simulink model "rhombus_vehicle_model_github"  (R2025b)
settings: Solver=VariableStepAuto  StartTime=0.0  StopTime=10.0  RelTol=1e-3
values from neighbouring files (symbols this model uses):
  B = 0.865    [vehicle_params_github.m]
  Bphi = 1.2e5    (= 120000)    [vehicle_params_github.m]
  Bx = 2    [vehicle_params_github.m]
  By = 1.5    [vehicle_params_github.m]
  Cw = 5    [vehicle_params_github.m]
  Cx = 1.1    [vehicle_params_github.m]
  Cy = 1.1    [vehicle_params_github.m]
  Ex = 0.3    [vehicle_params_github.m]
  Ey = -1.0    (= -1)    [vehicle_params_github.m]
  g = 9.81    [vehicle_params_github.m]
  hs = 1.25    [vehicle_params_github.m]
  Ix = 7.5e4    (= 75000)    [vehicle_params_github.m]
  Ixz = 0    [vehicle_params_github.m]
  Iz = 2.5e6    (= 2500000)    [vehicle_params_github.m]
  Jw = 60    [vehicle_params_github.m]
  kphi = 8e5    (= 800000)    [vehicle_params_github.m]
  lf = 4    [vehicle_params_github.m]
  lm = 0    [vehicle_params_github.m]
  lr = 4    [vehicle_params_github.m]
  m = 28000    [vehicle_params_github.m]
  ms = 22000    [vehicle_params_github.m]
  mux = 0.3    [vehicle_params_github.m]
  muy = 0.6    [vehicle_params_github.m]
  p = -0.15    [vehicle_params_github.m]
  Rw = 0.5    [vehicle_params_github.m]
settings Model: Creator=dastiw  LastModifiedBy=dastiw

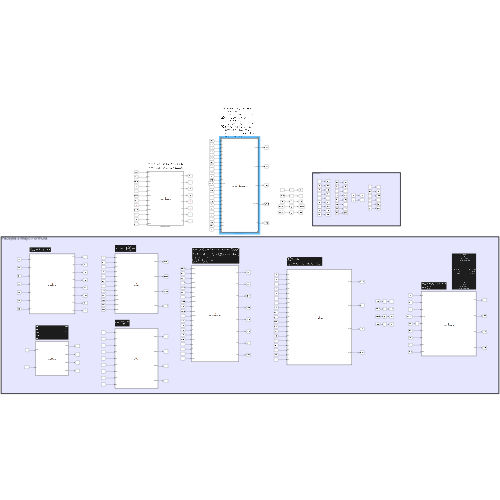
[thumbnail: Simulink's stored preview of the top-level diagram]
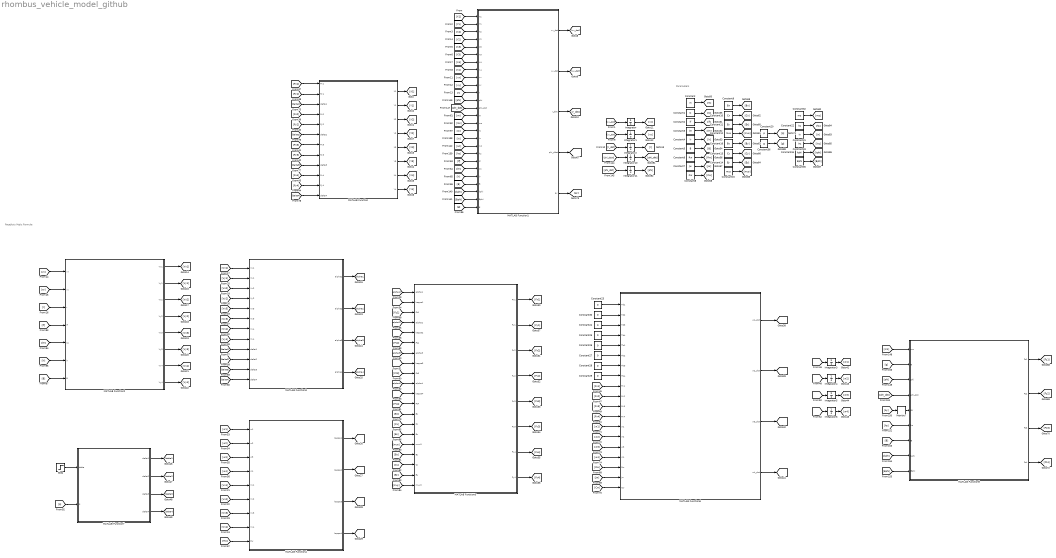
== system rhombus_vehicle_model_github ==
  note: Pacejka's Majic Formula
  note: Parameters
  Constant : Constant  Value=m
  Constant1 : Constant  Value=Iz
  Constant10 : Constant  Value=Cx
  Constant11 : Constant  Value=Ex
  Constant12 : Constant  Value=mux
  Constant13 : Constant  Value=Cy
  Constant14 : Constant  Value=Ey
  Constant15 : Constant  Value=muy
  Constant16 : Constant  Value=By
  Constant2 : Constant  Value=lf
  Constant20 : Constant  Value=p
  Constant22 : Constant  Value=hs
  Constant{23..30} (8 alike) : Constant  Value=0
  Constant3 : Constant  Value=lm
  Constant31 : Constant  Value=Ix
  Constant32 : Constant  Value=ms
  Constant33 : Constant  Value=Ixz
  Constant34 : Constant  Value=kphi
  Constant35 : Constant  Value=Bphi
  Constant36 : Constant  Value=g
  Constant4 : Constant  Value=lr
  Constant5 : Constant  Value=B
  Constant6 : Constant  Value=Rw
  Constant7 : Constant  Value=Jw
  Constant8 : Constant  Value=Cw
  Constant9 : Constant  Value=Bx
  Integrator : Integrator  InitialCondition=5
  Integrator{1..2,10..11} (4 alike) : Integrator
  Integrator{3..6} (4 alike) : Integrator  InitialCondition=5/Rw
  MATLAB Function : MATLAB Function  TreatAsAtomicUnit=on
  MATLAB Function1 : MATLAB Function  TreatAsAtomicUnit=on
  MATLAB Function2 : MATLAB Function  TreatAsAtomicUnit=on
  MATLAB Function3 : MATLAB Function  TreatAsAtomicUnit=on
  MATLAB Function4 : MATLAB Function  TreatAsAtomicUnit=on
  MATLAB Function5 : MATLAB Function  TreatAsAtomicUnit=on
  MATLAB Function6 : MATLAB Function  TreatAsAtomicUnit=on
  MATLAB Function7 : MATLAB Function  TreatAsAtomicUnit=on
  MATLAB Function9 : MATLAB Function  TreatAsAtomicUnit=on
  Memory : Memory
  Step : Step  After=0.01  SampleTime=0
  wires:
  MATLAB Function/1(X1) -> [X1]
  MATLAB Function/8(Y4) -> [Y4]
  MATLAB Function/2(Y1) -> [Y1]
  MATLAB Function/3(X2) -> [X2]
  MATLAB Function/4(Y2) -> [Y2]
  MATLAB Function/5(X3) -> [X3]
  MATLAB Function/6(Y3) -> [Y3]
  MATLAB Function/7(X4) -> [X4]
  MATLAB Function1/1(vx_dot) -> [vx_dot]
  MATLAB Function1/2(vy_dot) -> [vy_dot]
  MATLAB Function1/3(r_dot) -> [r_dot]
  [vx_dot] -> Integrator/1
  [vy_dot] -> Integrator1/1
  [r_dot] -> Integrator2/1
  Integrator/1 -> [vx]
  Integrator1/1 -> [vy]
  Integrator2/1 -> [r]
  [vy] -> MATLAB Function2/2(vy)
  [vx] -> MATLAB Function2/1(vx)
  [r] -> MATLAB Function2/3(r)
  MATLAB Function2/1(Vx1) -> [Vx1]
  MATLAB Function2/3(Vx2) -> [Vx2]
  MATLAB Function2/5(Vx3) -> [Vx3]
  MATLAB Function2/7(Vx4) -> [Vx4]
  [Vx1] -> MATLAB Function3/1(Vx1)
  [Vx2] -> MATLAB Function3/3(Vx2)
  [Vx3] -> MATLAB Function3/5(Vx3)
  [Vx4] -> MATLAB Function3/7(Vx4)
  [Vx1] -> MATLAB Function4/5(Vx1)
  [Vx4] -> MATLAB Function4/8(Vx4)
  [Vx3] -> MATLAB Function4/7(Vx3)
  [Vx2] -> MATLAB Function4/6(Vx2)
  MATLAB Function2/2(Vy1) -> [Vy1]
  MATLAB Function2/4(Vy2) -> [Vy2]
  MATLAB Function2/6(Vy3) -> [Vy3]
  MATLAB Function2/8(Vy4) -> [Vy4]
  [Vy1] -> MATLAB Function3/2(Vy1)
  [Vy2] -> MATLAB Function3/4(Vy2)
  [Vy3] -> MATLAB Function3/6(Vy3)
  [Vy4] -> MATLAB Function3/8(Vy4)
  MATLAB Function3/1(alpha1) -> [alpha1]
  MATLAB Function3/2(alpha2) -> [alpha2]
  MATLAB Function3/3(alpha3) -> [alpha3]
  MATLAB Function3/4(alpha4) -> [alpha4]
  MATLAB Function4/1(kappa1) -> [kappa1]
  MATLAB Function4/2(kappa2) -> [kappa2]
  MATLAB Function4/3(kappa3) -> [kappa3]
  MATLAB Function4/4(kappa4) -> [kappa4]
  [alpha1] -> MATLAB Function5/1(alpha1)
  [kappa1] -> MATLAB Function5/2(kappa1)
  [alpha2] -> MATLAB Function5/4(alpha2)
  [kappa2] -> MATLAB Function5/5(kappa2)
  [alpha3] -> MATLAB Function5/7(alpha3)
  [kappa3] -> MATLAB Function5/8(kappa3)
  [alpha4] -> MATLAB Function5/10(alpha4)
  [kappa4] -> MATLAB Function5/11(kappa4)
  MATLAB Function5/1(Fx1) -> [Fx1]
  MATLAB Function5/2(Fy1) -> [Fy1]
  MATLAB Function5/3(Fx2) -> [Fx2]
  MATLAB Function5/4(Fy2) -> [Fy2]
  MATLAB Function5/5(Fx3) -> [Fx3]
  MATLAB Function5/6(Fy3) -> [Fy3]
  MATLAB Function5/7(Fx4) -> [Fx4]
  MATLAB Function5/8(Fy4) -> [Fy4]
  [Fx1] -> MATLAB Function/1(Fx1)
  [Fy1] -> MATLAB Function/2(Fy1)
  [Fx2] -> MATLAB Function/4(Fx2)
  [Fy2] -> MATLAB Function/5(Fy2)
  [Fx3] -> MATLAB Function/7(Fx3)
  [Fy3] -> MATLAB Function/8(Fy3)
  [Fx4] -> MATLAB Function/10(Fx4)
  [Fy4] -> MATLAB Function/11(Fy4)
  [Fx1] -> MATLAB Function6/9(Fx1)
  [Fx2] -> MATLAB Function6/10(Fx2)
  [Fx3] -> MATLAB Function6/11(Fx3)
  [Fx4] -> MATLAB Function6/12(Fx4)
  MATLAB Function6/1(w1_dot) -> [w1_dot]
  MATLAB Function6/2(w2_dot) -> [w2_dot]
  MATLAB Function6/3(w3_dot) -> [w3_dot]
  MATLAB Function6/4(w4_dot) -> [w4_dot]
  [w1_dot] -> Integrator3/1
  [w4_dot] -> Integrator6/1
  [w3_dot] -> Integrator5/1
  [w2_dot] -> Integrator4/1
  Integrator3/1 -> [w1]
  Integrator6/1 -> [w4]
  Integrator5/1 -> [w3]
  Integrator4/1 -> [w2]
  [w1] -> MATLAB Function4/1(w1)
  [w2] -> MATLAB Function4/2(w2)
  [w3] -> MATLAB Function4/3(w3)
  [w4] -> MATLAB Function4/4(w4)
  MATLAB Function7/1(delta1) -> [delta1]
  MATLAB Function7/2(delta2) -> [delta2]
  MATLAB Function7/3(delta3) -> [delta3]
  MATLAB Function7/4(delta4) -> [delta4]
  [delta1] -> MATLAB Function3/9(delta1)
  [delta2] -> MATLAB Function3/10(delta2)
  [delta3] -> MATLAB Function3/11(delta3)
  [delta4] -> MATLAB Function3/12(delta4)
  [Rw] -> MATLAB Function4/9(Rw)
  [Rw] -> MATLAB Function6/17(Rw)
  [Cw] -> MATLAB Function6/19(Cw)
  [Jw] -> MATLAB Function6/18(Jw)
  [w3] -> MATLAB Function6/15(w3)
  [w2] -> MATLAB Function6/14(w2)
  [w1] -> MATLAB Function6/13(w1)
  [w4] -> MATLAB Function6/16(w4)
  [delta1] -> MATLAB Function/3(delta1)
  [delta2] -> MATLAB Function/6(delta2)
  [delta4] -> MATLAB Function/12(delta4)
  [delta3] -> MATLAB Function/9(delta3)
  [Bx] -> MATLAB Function5/13(Bx)
  [Cx] -> MATLAB Function5/14(Cx)
  [Ex] -> MATLAB Function5/15(Ex)
  [mux] -> MATLAB Function5/16(mux0)
  [By] -> MATLAB Function5/17(By)
  [Cy] -> MATLAB Function5/18(Cy)
  [Ey] -> MATLAB Function5/19(Ey)
  [muy] -> MATLAB Function5/20(muy0)
  [B] -> MATLAB Function2/7(B)
  [Fz1] -> MATLAB Function5/3(Fz1)
  [Fz2] -> MATLAB Function5/6(Fz2)
  [Fz3] -> MATLAB Function5/9(Fz3)
  [Fz4] -> MATLAB Function5/12(Fz4)
  [p] -> MATLAB Function7/2(p)
  [lf] -> MATLAB Function2/4(lf)
  [lm] -> MATLAB Function2/5(lm)
  [lr] -> MATLAB Function2/6(lr)
  Constant23/1 -> MATLAB Function6/1(Td1)
  Constant29/1 -> MATLAB Function6/8(Tb4)
  Constant28/1 -> MATLAB Function6/7(Tb3)
  Constant27/1 -> MATLAB Function6/6(Tb2)
  Constant26/1 -> MATLAB Function6/5(Tb1)
  Constant25/1 -> MATLAB Function6/4(Td4)
  Constant24/1 -> MATLAB Function6/3(Td3)
  Constant30/1 -> MATLAB Function6/2(Td2)
  Step/1 -> MATLAB Function7/1(delta)
  [X1] -> MATLAB Function1/1(X1)
  [Y1] -> MATLAB Function1/2(Y1)
  [X2] -> MATLAB Function1/3(X2)
  [Y2] -> MATLAB Function1/4(Y2)
  [X3] -> MATLAB Function1/5(X3)
  [Y3] -> MATLAB Function1/6(Y3)
  [X4] -> MATLAB Function1/7(X4)
  [Y4] -> MATLAB Function1/8(Y4)
  [vx] -> MATLAB Function1/9(vx)
  [vy] -> MATLAB Function1/10(vy)
  [r] -> MATLAB Function1/11(r)
  [m] -> MATLAB Function1/14(m)
  [ms] -> MATLAB Function1/15(ms)
  [lf] -> MATLAB Function1/20(lf)
  [lm] -> MATLAB Function1/21(lm)
  [lr] -> MATLAB Function1/22(lr)
  [B] -> MATLAB Function1/23(B)
  Constant10/1 -> [Cx]
  Constant9/1 -> [Bx]
  Constant12/1 -> [mux]
  Constant32/1 -> [ms]
  Constant16/1 -> [By]
  Constant13/1 -> [Cy]
  Constant20/1 -> [p]
  Constant14/1 -> [Ey]
  Constant33/1 -> [Ixz]
  Constant5/1 -> [B]
  Constant31/1 -> [Ix]
  Constant22/1 -> [hs]
  Constant/1 -> [m]
  Constant7/1 -> [Jw]
  Constant3/1 -> [lm]
  Constant4/1 -> [lr]
  Constant11/1 -> [Ex]
  Constant15/1 -> [muy]
  Constant34/1 -> [kphi]
  Constant35/1 -> [Bphi]
  Constant36/1 -> [g]
  Constant1/1 -> [Iz]
  Constant2/1 -> [lf]
  Constant8/1 -> [Cw]
  Constant6/1 -> [Rw]
  [Bphi] -> MATLAB Function1/25(Bphi)
  [kphi] -> MATLAB Function1/24(kphi)
  [g] -> MATLAB Function1/26(g)
  [Ixz] -> MATLAB Function1/18(Ixz)
  [Ix] -> MATLAB Function1/17(Ix)
  [Iz] -> MATLAB Function1/16(Iz)
  [hs] -> MATLAB Function1/19(hs)
  [phi_dot] -> MATLAB Function1/13(phi_dot)
  [phi] -> MATLAB Function1/12(phi)
  [phi_dot] -> Integrator11/1
  Integrator11/1 -> [phi]
  [phi_ddot] -> Integrator10/1
  Integrator10/1 -> [phi_dot]
  MATLAB Function1/4(phi_ddot) -> [phi_ddot]
  [ms] -> MATLAB Function9/1(ms)
  [g] -> MATLAB Function9/2(g)
  MATLAB Function9/2(Fz2) -> [Fz2]
  MATLAB Function9/4(Fz4) -> [Fz4]
  [phi] -> MATLAB Function9/3(phi)
  [B] -> MATLAB Function9/7(B)
  [Bphi] -> MATLAB Function9/9(Bphi)
  MATLAB Function9/1(Fz1) -> [Fz1]
  [hs] -> MATLAB Function9/6(hs)
  [kphi] -> MATLAB Function9/8(kphi)
  MATLAB Function9/3(Fz3) -> [Fz3]
  [phi_dot] -> MATLAB Function9/4(phi_dot)
  MATLAB Function1/5(ay) -> [ay]
  [ay] -> Memory/1
  Memory/1 -> MATLAB Function9/5(ay)

== matlab function rhombus_vehicle_model_github/MATLAB Function ==
  data: Fx1 input; X1 output; Fy1 input; delta1 input; Fx2 input; Fy2 input; delta2 input; Fx3 input; Fy3 input; delta3 input; Fx4 input; Fy4 input; delta4 input; Y1 output; X2 output; Y2 output; X3 output; Y3 output; X4 output; Y4 output
function [X1,Y1,X2,Y2,X3,Y3,X4,Y4] = ...
ForceTransformation( ...
Fx1,Fy1,delta1,...
Fx2,Fy2,delta2,...
Fx3,Fy3,delta3,...
Fx4,Fy4,delta4)

% Wheel 1
X1 = Fx1*cos(delta1) - Fy1*sin(delta1);
Y1 = Fx1*sin(delta1) + Fy1*cos(delta1);

% Wheel 2
X2 = Fx2*cos(delta2) - Fy2*sin(delta2);
Y2 = Fx2*sin(delta2) + Fy2*cos(delta2);

% Wheel 3
X3 = Fx3*cos(delta3) - Fy3*sin(delta3);
Y3 = Fx3*sin(delta3) + Fy3*cos(delta3);

% Wheel 4
X4 = Fx4*cos(delta4) - Fy4*sin(delta4);
Y4 = Fx4*sin(delta4) + Fy4*cos(delta4);

end

== matlab function rhombus_vehicle_model_github/MATLAB Function2 ==
  data: vx input; Vx1 output; vy input; r input; lf input; lm input; lr input; B input; Vy1 output; Vx2 output; Vy2 output; Vx3 output; Vy3 output; Vx4 output; Vy4 output
function [Vx1,Vy1,...
          Vx2,Vy2,...
          Vx3,Vy3,...
          Vx4,Vy4] = ...
WheelVelocities(vx,vy,r,lf,lm,lr,B)

% Front wheel
Vx1 = vx;
Vy1 = vy + r*lf;

% Middle-left wheel
Vx2 = vx - r*B;
Vy2 = vy - r*lm;

% Middle-right wheel
Vx3 = vx + r*B;
Vy3 = vy - r*lm;

% Rear wheel
Vx4 = vx;
Vy4 = vy - r*lr;

end

== matlab function rhombus_vehicle_model_github/MATLAB Function3 ==
  data: Vx1 input; alpha1 output; Vy1 input; Vx2 input; Vy2 input; Vx3 input; Vy3 input; Vx4 input; Vy4 input; delta1 input; delta2 input; delta3 input; delta4 input; alpha2 output; alpha3 output; alpha4 output
function [alpha1,alpha2,alpha3,alpha4] = ...
SlipAngles( ...
Vx1,Vy1,...
Vx2,Vy2,...
Vx3,Vy3,...
Vx4,Vy4,...
delta1,delta2,delta3,delta4)

eps_v = 0.1;

Vx1s = sign(Vx1)*max(abs(Vx1),eps_v);
Vx2s = sign(Vx2)*max(abs(Vx2),eps_v);
Vx3s = sign(Vx3)*max(abs(Vx3),eps_v);
Vx4s = sign(Vx4)*max(abs(Vx4),eps_v);

alpha1 = atan2(Vy1,Vx1s) - delta1;

alpha2 = atan2(Vy2,Vx2s) - delta2;

alpha3 = atan2(Vy3,Vx3s) - delta3;

alpha4 = atan2(Vy4,Vx4s) - delta4;

end

== matlab function rhombus_vehicle_model_github/MATLAB Function4 ==
  data: w1 input; kappa1 output; w2 input; w3 input; w4 input; Vx1 input; Vx2 input; Vx3 input; Vx4 input; Rw input; kappa2 output; kappa3 output; kappa4 output
function [kappa1,kappa2,kappa3,kappa4] = ...
SlipRatios( ...
w1,w2,w3,w4,...
Vx1,Vx2,Vx3,Vx4,...
Rw)

% Numerical protection threshold
eps_v = 1.0;

% Safe velocities
Vx1_safe = max(abs(Vx1),eps_v);
Vx2_safe = max(abs(Vx2),eps_v);
Vx3_safe = max(abs(Vx3),eps_v);
Vx4_safe = max(abs(Vx4),eps_v);

% Raw slip ratios
kappa1_raw = (Rw*w1 - Vx1) / Vx1_safe;
kappa2_raw = (Rw*w2 - Vx2) / Vx2_safe;
kappa3_raw = (Rw*w3 - Vx3) / Vx3_safe;
kappa4_raw = (Rw*w4 - Vx4) / Vx4_safe;

% Strong saturation for initial stability
kappa1 = max(min(kappa1_raw,0.1),-0.1);
kappa2 = max(min(kappa2_raw,0.1),-0.1);
kappa3 = max(min(kappa3_raw,0.1),-0.1);
kappa4 = max(min(kappa4_raw,0.1),-0.1);

end

== matlab function rhombus_vehicle_model_github/MATLAB Function5 ==
  data: alpha1 input; Fx1 output; kappa1 input; Fz1 input; alpha2 input; kappa2 input; Fz2 input; alpha3 input; kappa3 input; Fz3 input; alpha4 input; kappa4 input; Fz4 input; Bx input; Cx input; Ex input; mux0 input; By input; Cy input; Fy1 output; Fx2 output; Fy2 output; Fx3 output; Fy3 output; Fx4 output; Fy4 output; Ey input; muy0 input
function [Fx1,Fy1,...
          Fx2,Fy2,...
          Fx3,Fy3,...
          Fx4,Fy4] = ...
Pacejka4WheelModel( ...
alpha1,kappa1,Fz1,...
alpha2,kappa2,Fz2,...
alpha3,kappa3,Fz3,...
alpha4,kappa4,Fz4,...
Bx,Cx,Ex,mux0,...
By,Cy,Ey,muy0)

%% =====================================================
% REFERENCE LOAD
%% =====================================================

Fz_ref = 75000;

%% =====================================================
% NUMERICAL PROTECTION
%% =====================================================

Fz1 = max(Fz1,1000);
Fz2 = max(Fz2,1000);
Fz3 = max(Fz3,1000);
Fz4 = max(Fz4,1000);

%% =====================================================
% LOAD-SENSITIVE FRICTION
%% =====================================================

mux1 = mux0 * (Fz1/Fz_ref)^(-0.08);
mux2 = mux0 * (Fz2/Fz_ref)^(-0.08);
mux3 = mux0 * (Fz3/Fz_ref)^(-0.08);
mux4 = mux0 * (Fz4/Fz_ref)^(-0.08);

muy1 = muy0 * (Fz1/Fz_ref)^(-0.08);
muy2 = muy0 * (Fz2/Fz_ref)^(-0.08);
muy3 = muy0 * (Fz3/Fz_ref)^(-0.08);
muy4 = muy0 * (Fz4/Fz_ref)^(-0.08);

%% =====================================================
% PEAK FACTORS
%% =====================================================

Dx1 = mux1 * Fz1;
Dx2 = mux2 * Fz2;
Dx3 = mux3 * Fz3;
Dx4 = mux4 * Fz4;

Dy1 = muy1 * Fz1;
Dy2 = muy2 * Fz2;
Dy3 = muy3 * Fz3;
Dy4 = muy4 * Fz4;

%% =====================================================
% WHEEL 1
%% =====================================================

Bxk1 = Bx * kappa1;

Fx1 = Dx1 * sin( ...
    Cx * atan( ...
    Bxk1 - Ex*(Bxk1 - atan(Bxk1))));

Bya1 = By * alpha1;

Fy1 = Dy1 * sin( ...
    Cy * atan( ...
    Bya1 - Ey*(Bya1 - atan(Bya1))));

%% Friction ellipse

ellipse1 = ...
    (Fx1/(mux1*Fz1))^2 + ...
    (Fy1/(muy1*Fz1))^2;

if ellipse1 > 1

    scale1 = 1/sqrt(ellipse1);

    Fx1 = Fx1 * scale1;

    Fy1 = Fy1 * scale1;

end

%% =====================================================
% WHEEL 2
%% =====================================================

Bxk2 = Bx * kappa2;

Fx2 = Dx2 * sin( ...
    Cx * atan( ...
    Bxk2 - Ex*(Bxk2 - atan(Bxk2))));

Bya2 = By * alpha2;

Fy2 = Dy2 * sin( ...
    Cy * atan( ...
    Bya2 - Ey*(Bya2 - atan(Bya2))));

%% Friction ellipse

ellipse2 = ...
    (Fx2/(mux2*Fz2))^2 + ...
    (Fy2/(muy2*Fz2))^2;

if ellipse2 > 1

    scale2 = 1/sqrt(ellipse2);

    Fx2 = Fx2 * scale2;

    Fy2 = Fy2 * scale2;

end

%% =====================================================
% WHEEL 3
%% =====================================================

Bxk3 = Bx * kappa3;

Fx3 = Dx3 * sin( ...
    Cx * atan( ...
    Bxk3 - Ex*(Bxk3 - atan(Bxk3))));

Bya3 = By * alpha3;

Fy3 = Dy3 * sin( ...
    Cy * atan( ...
    Bya3 - Ey*(Bya3 - atan(Bya3))));

%% Friction ellipse

ellipse3 = ...
    (Fx3/(mux3*Fz3))^2 + ...
    (Fy3/(muy3*Fz3))^2;

if ellipse3 > 1

    scale3 = 1/sqrt(ellipse3);

    Fx3 = Fx3 * scale3;

    Fy3 = Fy3 * scale3;

end

%% =====================================================
% WHEEL 4
%% =====================================================

Bxk4 = Bx * kappa4;

Fx4 = Dx4 * sin( ...
    Cx * atan( ...
    Bxk4 - Ex*(Bxk4 - atan(Bxk4))));

Bya4 = By * alpha4;

Fy4 = Dy4 * sin( ...
    Cy * atan( ...
    Bya4 - Ey*(Bya4 - atan(Bya4))));

%% Friction ellipse

ellipse4 = ...
    (Fx4/(mux4*Fz4))^2 + ...
    (Fy4/(muy4*Fz4))^2;

if ellipse4 > 1

    scale4 = 1/sqrt(ellipse4);

    Fx4 = Fx4 * scale4;

    Fy4 = Fy4 * scale4;

end

end

== matlab function rhombus_vehicle_model_github/MATLAB Function6 ==
  data: Td1 input; w1_dot output; Td2 input; Td3 input; Td4 input; Tb1 input; Tb2 input; Tb3 input; Tb4 input; Fx1 input; Fx2 input; Fx3 input; Fx4 input; w1 input; w2 input; w3 input; w4 input; Rw input; Jw input; w2_dot output; w3_dot output; w4_dot output; Cw input
function [w1_dot,w2_dot,w3_dot,w4_dot] = ...
WheelDynamics( ...
Td1,Td2,Td3,Td4,...
Tb1,Tb2,Tb3,Tb4,...
Fx1,Fx2,Fx3,Fx4,...
w1,w2,w3,w4,...
Rw,Jw,Cw)

% Wheel rotational dynamics

% Wheel 1
Tw1 = Td1 - Tb1 - Rw*Fx1 - Cw*w1;
w1_dot = Tw1 / Jw;

% Wheel 2
Tw2 = Td2 - Tb2 - Rw*Fx2 - Cw*w2;
w2_dot = Tw2 / Jw;

% Wheel 3
Tw3 = Td3 - Tb3 - Rw*Fx3 - Cw*w3;
w3_dot = Tw3 / Jw;

% Wheel 4
Tw4 = Td4 - Tb4 - Rw*Fx4 - Cw*w4;
w4_dot = Tw4 / Jw;

end

== matlab function rhombus_vehicle_model_github/MATLAB Function7 ==
  data: delta input; delta1 output; p input; delta2 output; delta3 output; delta4 output
function [delta1,delta2,delta3,delta4] = ...
SteeringSystem(delta,p)

% Front steering
delta1 = delta;

% Middle wheels do not steer
delta2 = 0;

delta3 = 0;

% Rear steering
delta4 = p * delta;

end

== matlab function rhombus_vehicle_model_github/MATLAB Function9 ==
  data: ms input; Fz1 output; g input; phi input; phi_dot input; ay input; hs input; B input; kphi input; Bphi input; Fz2 output; Fz3 output; Fz4 output
function [Fz1,Fz2,Fz3,Fz4] = ...
DynamicVerticalLoads( ...
ms,g,...
phi,phi_dot,...
ay,...
hs,B,...
kphi,Bphi)

%% =====================================================
% STATIC LOADS
%% =====================================================

Fz1_static = 8000*g;

Fz2_static = 6000*g;

Fz3_static = 6000*g;

Fz4_static = 8000*g;

%% =====================================================
% ROLL MOMENT
%% =====================================================

Mx = ...
      ms * hs * g * phi ...
    - kphi * phi ...
    - Bphi * phi_dot;

%% =====================================================
% LOAD TRANSFER
%% =====================================================

dF = Mx / (2*B);

%% =====================================================
% RHOMBUS LOAD DISTRIBUTION
%% =====================================================

% Front and rear wheels are on centerline
% therefore they do not experience
% lateral load transfer

Fz1 = Fz1_static;

Fz4 = Fz4_static;

% Middle wheels carry lateral transfer

Fz2 = Fz2_static + dF;

Fz3 = Fz3_static - dF;

%% =====================================================
% NUMERICAL PROTECTION
%% =====================================================

Fz1 = max(Fz1,1000);

Fz2 = max(Fz2,1000);

Fz3 = max(Fz3,1000);

Fz4 = max(Fz4,1000);

end

== matlab function rhombus_vehicle_model_github/MATLAB Function1 ==
  data: vx_dot output; vy_dot output; r_dot output; phi_ddot output; X1 input; Y1 input; X2 input; Y2 input; X3 input; Y3 input; X4 input; Y4 input; vx input; vy input; r input; phi input; phi_dot input; m input; ms input; Iz input; Ix input; Ixz input; hs input; lf input; lm input; lr input; B input; kphi input; Bphi input; g input; ay output
function [vx_dot, vy_dot, r_dot, phi_ddot, ay] = ...
VehicleDynamicsNonlinear(X1, Y1, X2, Y2, X3, Y3, X4, Y4, vx, vy, r, phi, phi_dot, m, ms, Iz, Ix, Ixz, hs, lf, lm, lr, B, kphi, Bphi, g)

%% =====================================================
% RHOMBIC VEHICLE NONLINEAR DYNAMICS
%
% States:
% vx        = longitudinal velocity
% vy        = lateral velocity
% r         = yaw rate
% phi       = roll angle
% phi_dot   = roll rate
%
% Outputs:
% vx_dot
% vy_dot
% r_dot
% phi_ddot
%
% Based on:
% "Analysis of Steering Dynamics of Rhombic
% New Concept Car"
%% =====================================================

%% =====================================================
% TOTAL FORCES
%% =====================================================

Fx_total = X1 + X2 + X3 + X4;

Fy_total = Y1 + Y2 + Y3 + Y4;

%% =====================================================
% YAW MOMENT
%% =====================================================

Mz = ...
      Y1 * lf ...
    - (Y2 + Y3) * lm ...
    + Y4 * lr ...
    + B * (X2 - X3);

%% =====================================================
% ROLL MOMENT
%% =====================================================

Mx = ...
      ms * hs * g * phi ...
    - kphi * phi ...
    - Bphi * phi_dot;

%% =====================================================
% COUPLED DYNAMICS MATRIX
%
% Unknowns:
% [ vy_dot
%   r_dot
%   phi_ddot ]
%% =====================================================

A_mat = [

      m,          0,          ms * hs;

      0,           Iz,        -Ixz;

      ms * hs,    -Ixz,        Ix

];

%% =====================================================
% RIGHT-HAND SIDE VECTOR
%% =====================================================

b_vec = [

    Fy_total + m * r * vx;

    Mz;

    Mx - ms * hs * r * vx

];

%% =====================================================
% SOLVE COUPLED EQUATIONS
%% =====================================================

solution = A_mat \ b_vec;

vy_dot   = solution(1);

r_dot    = solution(2);

phi_ddot = solution(3);

%% =====================================================
% LONGITUDINAL DYNAMICS
%
% m*(vx_dot - r*vy) - ms*hs*phi_dot*r = Fx_total
%% =====================================================

vx_dot = ...
    (Fx_total + ms * hs * phi_dot * r)/m ...
    + r * vy;

%% =====================================================
% LATERAL ACCELERATION
%% =====================================================

ay = vy_dot + r*vx;

end
